simulink model "sampleModel1651"  (R2023a)
settings: Solver=VariableStepAuto  StartTime=0.0  StopTime=10.0  RelTol=1e-3
libraries: simulink x3, hdlsllib x3
settings Model: Creator=user1  LastModifiedBy=user1

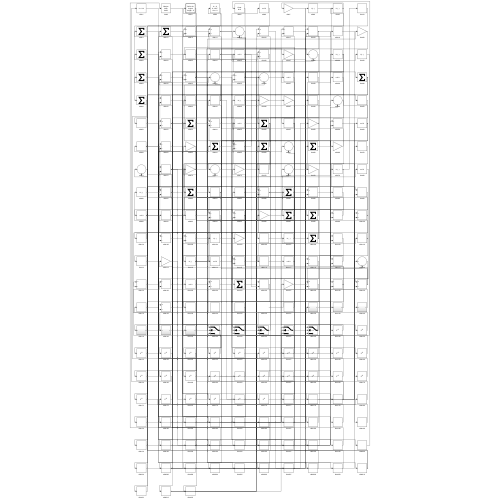
[thumbnail: Simulink's stored preview of the top-level diagram]
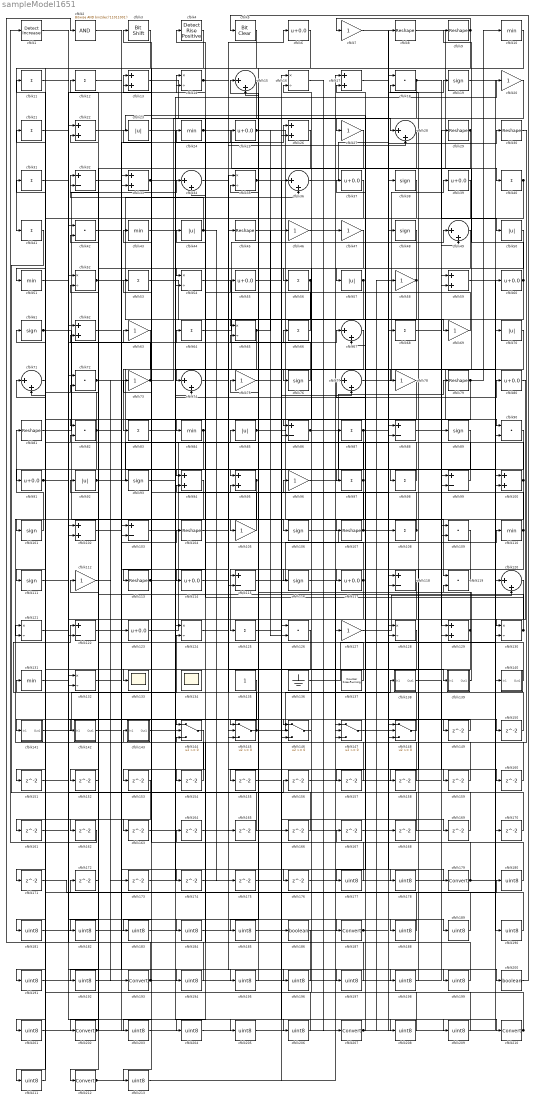
== system sampleModel1651 ==
  cfblk1 : simulink/Logic and Bit Operations/Detect Increase  vinit=0.0  OutDataTypeStr=boolean
      settings: LibrarySourceBlock=|
      | hdlsllib/Logic and Bit
      | Operations/Detect
      | Increase
  cfblk{10,24,43,51,84,110,131} (7 alike) : MinMax
  cfblk{13,17,22,26,33,59,62,94..95,100,102,129} (12 alike) : Sum
  cfblk{19,38,48,61,76,89,93,101,106,111,116} (11 alike) : Signum
  cfblk{32,86,88,99,103,115,118,122} (8 alike) : Sum  Inputs=+-
  cfblk{8..9,29..30,45,79,81,104,107,113} (10 alike) : Reshape
  cfblk{7,20,27,46..47,58,63,69,73,75,78,96,105,112,127} (15 alike) : Gain
  cfblk{11..12,21,31,40..41,53,56,64,66,68,83,87,97..98,108,125} (17 alike) : Sum  Inputs=+
  cfblk{18,42,72,82,90,109,119,126} (8 alike) : DotProduct  OutDataTypeStr=Inherit: Inherit via internal rule
  cfblk{6,25,37,39,55,60,80,91,114,117,123} (11 alike) : Bias  Bias=0.0  SaturateOnIntegerOverflow=off
  cfblk{15,28,34,36,49,67,71,74,77,120} (10 alike) : Sum  Inputs=|++
  cfblk{14,16,35,52,54,65,121,124,128,130,132} (11 alike) : Product  Inputs=*/  RndMeth=Zero  SaturateOnIntegerOverflow=on
  cfblk133 : Scope
  cfblk134 : Scope
      settings: Floating=on
  cfblk135 : Constant  SampleTime=-1
  cfblk136 : Ground
  cfblk137 : hdlsllib/Sources/Counter Free-Running  NumBits=16  tsamp=-1
  cfblk138 : Subsystem
      settings: LibrarySourceBlock=|
      | hdlsllib/Ports &
      | Subsystems/Subsystem
  cfblk139 : Subsystem
      settings: LibrarySourceBlock=|
      | hdlsllib/Ports &
      | Subsystems/Subsystem
  cfblk140 : Subsystem
      settings: LibrarySourceBlock=|
      | hdlsllib/Ports &
      | Subsystems/Subsystem
  cfblk141 : Subsystem
      settings: LibrarySourceBlock=|
      | hdlsllib/Ports &
      | Subsystems/Subsystem
  cfblk142 : Subsystem
      settings: LibrarySourceBlock=|
      | hdlsllib/Ports &
      | Subsystems/Subsystem
  cfblk143 : Subsystem
      settings: LibrarySourceBlock=|
      | hdlsllib/Ports &
      | Subsystems/Subsystem
  cfblk{144..148} (5 alike) : Switch  SaturateOnIntegerOverflow=off  InputSameDT=off
  cfblk{149..176} (28 alike) : Delay  SampleTime=1
  cfblk{177..178,180..185,188..192,194..199,201,203..206,208..209,211,213} (28 alike) : DataTypeConversion  OutDataTypeStr=uint8  SaturateOnIntegerOverflow=off  RndMeth=Floor
  cfblk{179,187,193,202,207,210,212} (7 alike) : DataTypeConversion  SaturateOnIntegerOverflow=off  RndMeth=Floor
  cfblk186 : DataTypeConversion  OutDataTypeStr=boolean  SaturateOnIntegerOverflow=off  RndMeth=Floor
  cfblk2 : simulink/Logic and Bit Operations/Bitwise Operator  logicop=AND  UseBitMask=on  BitMask=bin2dec('11011001')  BitMaskRealWorld=Stored Integer
      settings: LibrarySourceBlock=|
      | hdlsllib/Logic and Bit
      | Operations/Bitwise
      | Operator
  cfblk200 : DataTypeConversion  OutDataTypeStr=boolean  SaturateOnIntegerOverflow=off  RndMeth=Floor
  cfblk{23,44,50,57,70,85,92} (7 alike) : Abs  SaturateOnIntegerOverflow=off
  cfblk3 : hdlsllib/Logic and Bit Operations/Bit Shift  mode=Shift Left Logical  N=0
  cfblk4 : hdlsllib/Logic and Bit Operations/Detect Rise Positive  vinit=0  OutDataTypeStr=boolean
  cfblk5 : simulink/Logic and Bit Operations/Bit Clear  iBit=0
      settings: LibrarySourceBlock=|
      | hdlsllib/Logic and Bit
      | Operations/Bit Clear
  wires:
  cfblk101/1 -> cfblk81/1
  cfblk123/1 -> cfblk85/1
  cfblk107/1 -> cfblk24/1, cfblk30/1
  cfblk9/1 -> cfblk7/1, cfblk111/1
  cfblk106/1 -> cfblk110/1
  cfblk73/1 -> cfblk27/1, cfblk32/1
  cfblk25/1 -> cfblk107/1, cfblk126/2
  cfblk22/1 -> cfblk57/1
  cfblk77/1 -> cfblk39/1
  cfblk79/1 -> cfblk10/1, cfblk211/1
  cfblk148/1 -> cfblk122/1
  cfblk145/1 -> cfblk138/1(In1), cfblk95/2, cfblk43/1
  cfblk84/1 -> cfblk4/1, cfblk152/1
  cfblk16/1 -> cfblk207/1
  cfblk61/1 -> cfblk106/1, cfblk145/3
  cfblk57/1 -> cfblk154/1, cfblk204/1
  cfblk135/1 -> cfblk141/1(In1)
  cfblk147/1 -> cfblk179/1
  cfblk137/1 -> cfblk92/1
  cfblk63/1 -> cfblk94/1
  cfblk17/1 -> cfblk148/1
  cfblk53/1 -> cfblk69/1
  cfblk8/1 -> cfblk90/1
  cfblk80/1 -> cfblk130/1
  cfblk35/1 -> cfblk119/1, cfblk209/1
  cfblk6/1 -> cfblk105/1
  cfblk103/1 -> cfblk96/1
  cfblk81/1 -> cfblk34/1
  cfblk65/1 -> cfblk83/1, cfblk46/1
  cfblk87/1 -> cfblk48/1, cfblk102/2
  cfblk47/1 -> cfblk212/1
  cfblk92/1 -> cfblk38/1, cfblk146/1
  cfblk13/1 -> cfblk28/1
  cfblk130/1 -> cfblk72/2, cfblk44/1
  cfblk46/1 -> cfblk17/1
  cfblk128/1 -> cfblk202/1
  cfblk108/1 -> cfblk75/1, cfblk94/2
  cfblk26/1 -> cfblk33/2
  cfblk54/1 -> cfblk130/2
  cfblk96/1 -> cfblk79/1
  cfblk64/1 -> cfblk49/1
  cfblk30/1 -> cfblk143/1(In1)
  cfblk24/1 -> cfblk40/1, cfblk28/2
  cfblk72/1 -> cfblk140/1(In1), cfblk22/2, cfblk173/1, cfblk174/1
  cfblk95/1 -> cfblk101/1, cfblk161/1
  cfblk112/1 -> cfblk193/1
  cfblk76/1 -> cfblk15/1
  cfblk113/1 -> cfblk68/1, cfblk80/1, cfblk208/1
  cfblk3/1 -> cfblk41/1
  cfblk32/1 -> cfblk144/1
  cfblk37/1 -> cfblk144/2
  cfblk91/1 -> cfblk64/1, cfblk14/2
  cfblk110/1 -> cfblk53/1, cfblk158/1
  cfblk114/1 -> cfblk45/1
  cfblk121/1 -> cfblk52/1
  cfblk85/1 -> cfblk129/1, cfblk145/1
  cfblk143/1(Out1) -> cfblk124/1
  cfblk33/1 -> cfblk78/1, cfblk74/2
  cfblk115/1 -> cfblk8/1
  cfblk58/1 -> cfblk56/1, cfblk97/1
  cfblk11/1 -> cfblk122/2
  cfblk141/1(Out1) -> cfblk124/2
  cfblk2/1 -> cfblk187/1
  cfblk102/1 -> cfblk26/1
  cfblk68/1 -> cfblk29/1
  cfblk109/1 -> cfblk125/1
  cfblk129/1 -> cfblk35/2, cfblk203/1
  cfblk42/1 -> cfblk123/1
  cfblk98/1 -> cfblk21/1
  cfblk20/1 -> cfblk113/1
  cfblk146/1 -> cfblk66/1
  cfblk136/1 -> cfblk120/1
  cfblk27/1 -> cfblk65/1
  cfblk90/1 -> cfblk117/1
  cfblk99/1 -> cfblk73/1
  cfblk139/1(Out1) -> cfblk119/2
  cfblk60/1 -> cfblk9/1, cfblk109/2, cfblk74/1
  cfblk14/1 -> cfblk6/1, cfblk200/1
  cfblk28/1 -> cfblk142/1(In1)
  cfblk50/1 -> cfblk114/1
  cfblk119/1 -> cfblk116/1
  cfblk36/1 -> cfblk19/1
  cfblk4/1 -> cfblk133/1
  cfblk66/1 -> cfblk55/1
  cfblk93/1 -> cfblk20/1
  cfblk15/1 -> cfblk54/1
  cfblk117/1 -> cfblk14/1, cfblk155/1
  cfblk7/1 -> cfblk108/1
  cfblk86/1 -> cfblk98/1, cfblk87/1
  cfblk44/1 -> cfblk32/2, cfblk13/2, cfblk175/1
  cfblk49/1 -> cfblk76/1
  cfblk56/1 -> cfblk86/1, cfblk146/3
  cfblk82/1 -> cfblk11/1, cfblk115/2, cfblk191/1
  cfblk18/1 -> cfblk115/1, cfblk50/1
  cfblk52/1 -> cfblk89/1, cfblk36/2
  cfblk78/1 -> cfblk91/1
  cfblk38/1 -> cfblk51/1
  cfblk132/1 -> cfblk93/1
  cfblk140/1(Out1) -> cfblk37/1
  cfblk105/1 -> cfblk3/1
  cfblk48/1 -> cfblk84/1
  cfblk131/1 -> cfblk210/1
  cfblk40/1 -> cfblk71/2, cfblk182/1
  cfblk124/1 -> cfblk139/1(In1)
  cfblk69/1 -> cfblk34/2
  cfblk100/1 -> cfblk17/2, cfblk121/2
  cfblk23/1 -> cfblk95/1
  cfblk55/1 -> cfblk77/2
  cfblk97/1 -> cfblk13/1, cfblk145/2, cfblk23/1
  cfblk83/1 -> cfblk100/2
  cfblk127/1 -> cfblk120/2
  cfblk88/1 -> cfblk99/2
  cfblk111/1 -> cfblk67/1
  cfblk122/1 -> cfblk104/1
  cfblk120/1 -> cfblk132/2
  cfblk29/1 -> cfblk82/1, cfblk148/3
  cfblk104/1 -> cfblk149/1
  cfblk149/1 -> cfblk148/2
  cfblk116/1 -> cfblk150/1
  cfblk150/1 -> cfblk35/1
  cfblk71/1 -> cfblk151/1
  cfblk144/1 -> cfblk153/1
  cfblk154/1 -> cfblk121/1
  cfblk41/1 -> cfblk156/1
  cfblk156/1 -> cfblk129/2
  cfblk39/1 -> cfblk157/1
  cfblk157/1 -> cfblk15/2
  cfblk158/1 -> cfblk103/1
  cfblk34/1 -> cfblk159/1
  cfblk159/1 -> cfblk33/1
  cfblk138/1(Out1) -> cfblk160/1
  cfblk160/1 -> cfblk65/2
  cfblk161/1 -> cfblk132/1
  cfblk94/1 -> cfblk162/1
  cfblk162/1 -> cfblk1/1
  cfblk67/1 -> cfblk163/1
  cfblk163/1 -> cfblk88/2
  cfblk74/1 -> cfblk165/1
  cfblk165/1 -> cfblk22/1
  cfblk166/1 -> cfblk72/1
  cfblk167/1 -> cfblk49/2
  cfblk168/1 -> cfblk82/2
  cfblk45/1 -> cfblk169/1
  cfblk169/1 -> cfblk99/1
  cfblk19/1 -> cfblk170/1
  cfblk170/1 -> cfblk102/1
  cfblk126/1 -> cfblk171/1
  cfblk172/1 -> cfblk52/2
  cfblk173/1 -> cfblk54/2
  cfblk174/1 -> cfblk86/2
  cfblk175/1 -> cfblk26/2
  cfblk142/1(Out1) -> cfblk176/1
  cfblk176/1 -> cfblk100/1
  cfblk70/1 -> cfblk177/1
  cfblk177/1 -> cfblk63/1
  cfblk75/1 -> cfblk178/1
  cfblk178/1 -> cfblk70/1
  cfblk179/1 -> cfblk90/2, cfblk144/3, cfblk88/1
  cfblk171/1 -> cfblk180/1
  cfblk180/1 -> cfblk147/1
  cfblk153/1 -> cfblk181/1
  cfblk181/1 -> cfblk147/2
  cfblk182/1 -> cfblk147/3
  cfblk118/1 -> cfblk183/1
  cfblk183/1 -> cfblk127/1
  cfblk151/1 -> cfblk184/1
  cfblk184/1 -> cfblk118/1
  cfblk89/1 -> cfblk185/1
  cfblk185/1 -> cfblk118/2
  cfblk186/1 -> cfblk2/1
  cfblk187/1 -> cfblk168/1, cfblk167/1
  cfblk12/1 -> cfblk188/1
  cfblk188/1 -> cfblk71/1
  cfblk21/1 -> cfblk189/1
  cfblk189/1 -> cfblk12/1
  cfblk59/1 -> cfblk190/1
  cfblk190/1 -> cfblk42/2
  cfblk191/1 -> cfblk59/1
  cfblk152/1 -> cfblk192/1
  cfblk192/1 -> cfblk59/2
  cfblk193/1 -> cfblk109/1, cfblk42/1
  cfblk51/1 -> cfblk194/1
  cfblk194/1 -> cfblk112/1
  cfblk62/1 -> cfblk195/1
  cfblk195/1 -> cfblk25/1
  cfblk1/1 -> cfblk196/1
  cfblk196/1 -> cfblk62/1
  cfblk155/1 -> cfblk197/1
  cfblk197/1 -> cfblk62/2
  cfblk164/1 -> cfblk198/1
  cfblk198/1 -> cfblk18/2
  cfblk125/1 -> cfblk199/1
  cfblk199/1 -> cfblk164/1
  cfblk200/1 -> cfblk5/1
  cfblk5/1 -> cfblk201/1
  cfblk201/1 -> cfblk103/2
  cfblk202/1 -> cfblk172/1, cfblk126/1, cfblk36/1, cfblk18/1
  cfblk203/1 -> cfblk128/1
  cfblk204/1 -> cfblk128/2
  cfblk31/1 -> cfblk205/1
  cfblk205/1 -> cfblk60/1
  cfblk43/1 -> cfblk206/1
  cfblk206/1 -> cfblk31/1
  cfblk207/1 -> cfblk67/2, cfblk58/1
  cfblk208/1 -> cfblk16/1
  cfblk209/1 -> cfblk16/2
  cfblk210/1 -> cfblk61/1, cfblk77/1
  cfblk211/1 -> cfblk131/1
  cfblk212/1 -> cfblk186/1, cfblk166/1, cfblk146/2
  cfblk10/1 -> cfblk213/1
  cfblk213/1 -> cfblk47/1

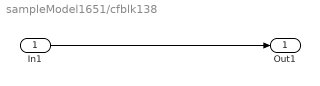
== system sampleModel1651/cfblk138 ==
  In1 : Inport
  Out1 : Outport
  wires:
  In1/1 -> Out1/1

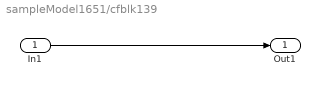
== system sampleModel1651/cfblk139 ==
  In1 : Inport
  Out1 : Outport
  wires:
  In1/1 -> Out1/1

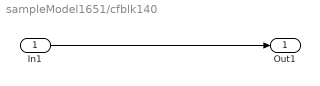
== system sampleModel1651/cfblk140 ==
  In1 : Inport
  Out1 : Outport
  wires:
  In1/1 -> Out1/1

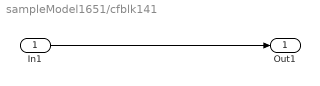
== system sampleModel1651/cfblk141 ==
  In1 : Inport
  Out1 : Outport
  wires:
  In1/1 -> Out1/1

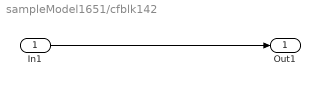
== system sampleModel1651/cfblk142 ==
  In1 : Inport
  Out1 : Outport
  wires:
  In1/1 -> Out1/1

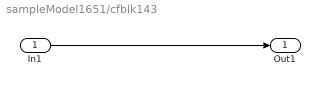
== system sampleModel1651/cfblk143 ==
  In1 : Inport
  Out1 : Outport
  wires:
  In1/1 -> Out1/1
